simulink model "InverseDynamicsControl"  (R2020b)
settings: Solver=VariableStepAuto  StartTime=0.0  StopTime=10.0  RelTol=1e-3
undefined symbols (not defined in the file): a0, a1, a2, a3, a_2, d_10, g, Il_2, Im_1, Im_2, k_d, k_p, kr_1, kr_2, l_2, ml_1, ml_2, mm_1, theta_20
libraries: simulink x1
settings Model: Creator=Musta  LastModifiedBy=Musta

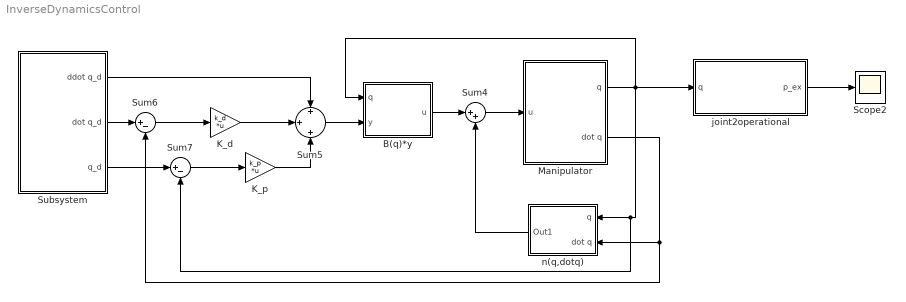
== system InverseDynamicsControl ==
  B(q)*y : Subsystem
  K_d : Gain  Gain=k_d  Multiplication=Matrix(K*u)
  K_p : Gain  Gain=k_p  Multiplication=Matrix(K*u)
  Manipulator : Subsystem
  Scope2 : Scope
  Subsystem : Subsystem
  Sum4 : Sum  Inputs=|++
  Sum5 : Sum  Inputs=+|+|+
  Sum6 : Sum  Inputs=|+-
  Sum7 : Sum  Inputs=|+-
  joint2operational : Subsystem
  n(q,dotq) : Subsystem
  wires:
  K_p/1 -> Sum5/3
  Manipulator/1(q) -> B(q)*y/1(q), joint2operational/1(q), n(q,dotq)/1(q), Sum7/2
  Sum4/1 -> Manipulator/1(u)
  Subsystem/1(ddot q_d) -> Sum5/1
  Subsystem/3(q_d) -> Sum7/1
  B(q)*y/1(u) -> Sum4/1
  joint2operational/1(p_ex) -> Scope2/1
  Sum6/1 -> K_d/1
  K_d/1 -> Sum5/2
  Sum7/1 -> K_p/1
  Subsystem/2(dot q_d) -> Sum6/1
  Manipulator/2(dot q) -> n(q,dotq)/2(dot q), Sum6/2
  Sum5/1 -> B(q)*y/2(y)
  n(q,dotq)/1(Out1) -> Sum4/2

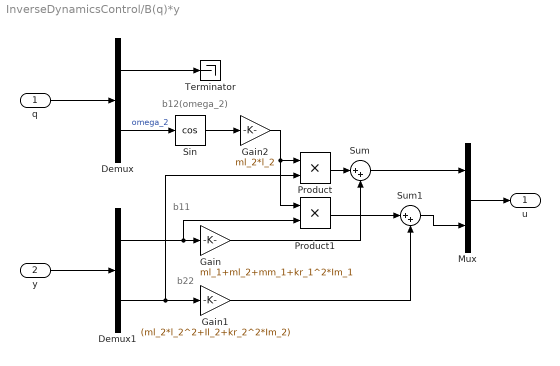
== system InverseDynamicsControl/B(q)*y ==
  note: b11
  note: b22
  note: b12(omega_2)
  q : Inport
  y : Inport  Port=2
  Demux : Demux  Outputs=2
  Demux1 : Demux  Outputs=2
  Gain : Gain  Gain=ml_1+ml_2+mm_1+kr_1^2*Im_1
  Gain1 : Gain  Gain=(ml_2*l_2^2+Il_2+kr_2^2*Im_2)
  Gain2 : Gain  Gain=ml_2*l_2
  Mux : Mux  Inputs=2
  Product : Product
  Product1 : Product
  Sin : Trigonometry  Operator=cos
  Sum : Sum  Inputs=|++
  Sum1 : Sum  Inputs=|++
  Terminator : Terminator
  u : Outport
  wires:
  Sum/1 -> Mux/1
  y/1 -> Demux1/1
  Mux/1 -> u/1
  Gain/1 -> Sum/2
  Demux1/1 -> Product1/2, Gain/1
  Demux/1 -> Terminator/1
  Gain2/1 -> Product1/1, Product/1
  Sin/1 -> Gain2/1
  Demux/2 -> Sin/1  "omega_2"
  Product/1 -> Sum/1
  Demux1/2 -> Product/2, Gain1/1
  q/1 -> Demux/1
  Gain1/1 -> Sum1/2
  Sum1/1 -> Mux/2
  Product1/1 -> Sum1/1

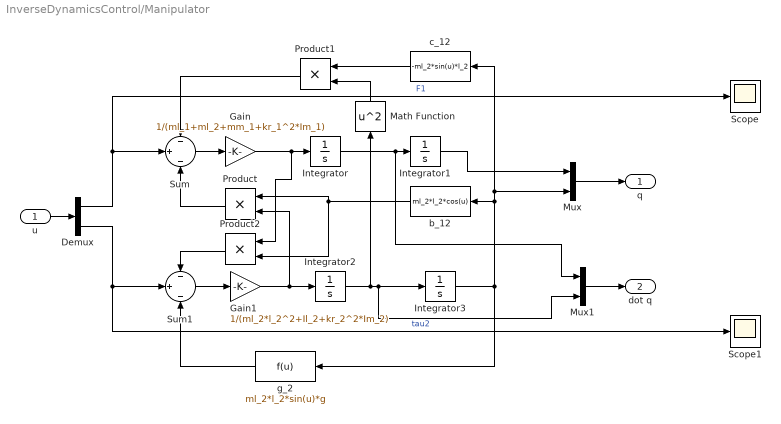
== system InverseDynamicsControl/Manipulator ==
  u : Inport
  Demux : Demux  Outputs=2
  Gain : Gain  Gain=1/(ml_1+ml_2+mm_1+kr_1^2*Im_1)
  Gain1 : Gain  Gain=1/(ml_2*l_2^2+Il_2+kr_2^2*Im_2)
  Integrator : Integrator
  Integrator1 : Integrator  InitialCondition=d_10
  Integrator2 : Integrator
  Integrator3 : Integrator  InitialCondition=theta_20
  Math Function : Math  Operator=square  SaturateOnIntegerOverflow=on
  Mux : Mux  Inputs=2
  Mux1 : Mux  Inputs=2
  Product : Product
  Product1 : Product
  Product2 : Product
  Scope : Scope
  Scope1 : Scope
  Sum : Sum  Inputs=-|+|-
  Sum1 : Sum  Inputs=-|+|-
  b_12 : Fcn  Expr=ml_2*l_2*cos(u)
  c_12 : Fcn  Expr=-ml_2*sin(u)*l_2
  g_2 : Fcn  Expr=ml_2*l_2*sin(u)*g
  q : Outport
  dot q : Outport  Port=2
  wires:
  Integrator2/1 -> Math Function/1, Mux1/2, Integrator3/1
  Integrator/1 -> Mux1/1, Integrator1/1
  Product/1 -> Sum/3
  Integrator1/1 -> Mux/1
  Mux/1 -> q/1
  b_12/1 -> Product2/2, Product/1
  Integrator3/1 -> c_12/1, Mux/2, b_12/1, g_2/1
  Sum1/1 -> Gain1/1
  Demux/1 -> Sum/2, Scope/1  "F1"
  Math Function/1 -> Product1/2
  Product2/1 -> Sum1/1
  c_12/1 -> Product1/1
  Product1/1 -> Sum/1
  Sum/1 -> Gain/1
  g_2/1 -> Sum1/3
  u/1 -> Demux/1
  Gain/1 -> Product2/1, Integrator/1
  Mux1/1 -> dot q/1
  Demux/2 -> Scope1/1, Sum1/2  "tau2"
  Gain1/1 -> Product/2, Integrator2/1

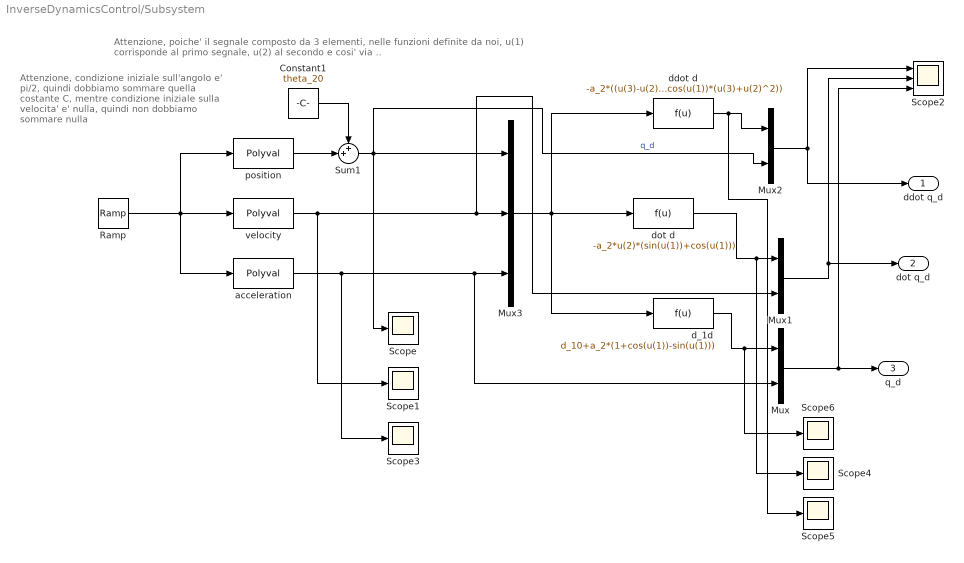
== system InverseDynamicsControl/Subsystem ==
  note: Attenzione, poiche' il segnale composto da 3 elementi, nelle funzioni definite da noi, u(1) corrisponde al primo segnale, u(2) al secondo e cosi' via ..
  note: Attenzione, condizione iniziale sull'angolo e' pi/2, quindi dobbiamo sommare quella costante C, mentre condizione iniziale sulla velocita' e' nulla, quindi non dobbiamo sommare nulla
  Constant1 : Constant  Value=theta_20
  Mux : Mux  Inputs=2
  Mux1 : Mux  Inputs=2
  Mux2 : Mux  Inputs=2
  Mux3 : Mux  Inputs=3
  Ramp : simulink/Sources/Ramp  slope=1  start=0  InitialOutput=0
  Scope{,1,3..6} (6 alike) : Scope
  Scope2 : Scope  NumInputPorts=3
  Sum1 : Sum  Inputs=++|
  acceleration : Polyval  Coefs=[6*a3, 2*a2]
  d_1d : Fcn  Expr=d_10+a_2*(1+cos(u(1))-sin(u(1)))
  ddot d : Fcn  Expr=-a_2*((u(3)-u(2)^2)*sin(u(1))+cos(u(1))*(u(3)+u(2)^2))
  dot d : Fcn  Expr=-a_2*u(2)*(sin(u(1))+cos(u(1)))
  position : Polyval  Coefs=[a3, a2, a1, a0]
  velocity : Polyval  Coefs=[3*a3, 2*a2, a1]
  ddot q_d : Outport
  dot q_d : Outport  Port=2
  q_d : Outport  Port=3
  wires:
  dot d/1 -> Scope4/1, Mux1/1
  Mux1/1 -> dot q_d/1, Scope2/2
  Mux/1 -> q_d/1, Scope2/3
  Mux3/1 -> d_1d/1, dot d/1, ddot d/1
  d_1d/1 -> Scope6/1, Mux/1
  ddot d/1 -> Scope5/1, Mux2/1
  Mux2/1 -> ddot q_d/1, Scope2/1
  Ramp/1 -> acceleration/1, velocity/1, position/1
  position/1 -> Sum1/2
  velocity/1 -> Scope1/1, Mux1/2, Mux3/2
  acceleration/1 -> Scope3/1, Mux/2, Mux3/3
  Constant1/1 -> Sum1/1
  Sum1/1 -> Mux2/2, Scope/1, Mux3/1  "q_d"

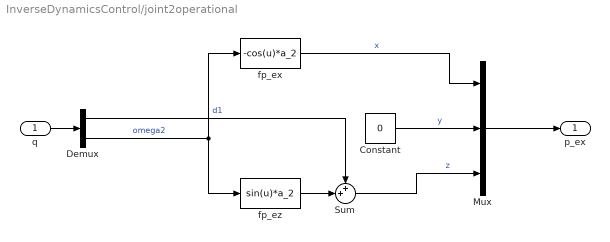
== system InverseDynamicsControl/joint2operational ==
  q : Inport
  Constant : Constant  Value=0
  Demux : Demux  Outputs=2
  Mux : Mux  Inputs=3
  Sum : Sum  Inputs=++|
  fp_ex : Fcn  Expr=-cos(u)*a_2
  fp_ez : Fcn  Expr=sin(u)*a_2
  p_ex : Outport
  wires:
  fp_ex/1 -> Mux/1  "x"
  Constant/1 -> Mux/2  "y"
  Demux/2 -> fp_ez/1, fp_ex/1  "omega2"
  Sum/1 -> Mux/3  "z"
  q/1 -> Demux/1
  fp_ez/1 -> Sum/2
  Demux/1 -> Sum/1  "d1"
  Mux/1 -> p_ex/1

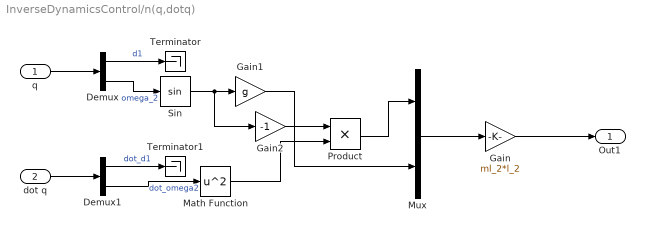
== system InverseDynamicsControl/n(q,dotq) ==
  q : Inport
  dot q : Inport  Port=2
  Demux : Demux  Outputs=2
  Demux1 : Demux  Outputs=2
  Gain : Gain  Gain=ml_2*l_2
  Gain1 : Gain  Gain=g
  Gain2 : Gain  Gain=-1
  Math Function : Math  Operator=square  SaturateOnIntegerOverflow=on
  Mux : Mux  Inputs=2
  Product : Product
  Sin : Trigonometry
  Terminator : Terminator
  Terminator1 : Terminator
  Out1 : Outport
  wires:
  Gain2/1 -> Product/1
  Demux1/2 -> Math Function/1  "dot_omega2"
  Demux/1 -> Terminator/1  "d1"
  Mux/1 -> Gain/1
  Demux/2 -> Sin/1  "omega_2"
  Gain/1 -> Out1/1
  Demux1/1 -> Terminator1/1  "dot_d1"
  Sin/1 -> Gain2/1, Gain1/1
  Product/1 -> Mux/1
  q/1 -> Demux/1
  dot q/1 -> Demux1/1
  Gain1/1 -> Mux/2
  Math Function/1 -> Product/2
